simulink model "FLPD"  (R2024b)
settings: Solver=ode45  StartTime=0.0  StopTime=20  MinStep=0.00002  RelTol=1e-9
InitFcn:
  | addpath('./../Robot Description/Robot Data Package/meshes/visual/')
  | addpath('./../Dynamics and Kinematics/')
  | 
  | % Controller Design
  | Design;
values from neighbouring files (symbols this model uses):
  Kd = 100000    [Design.m]
  Kp = 100000    [Design.m]
  qInitDM = [zeros(14, 1)]    [Design.m]
settings Model: Creator=Banaan  LastModifiedBy=Banaan

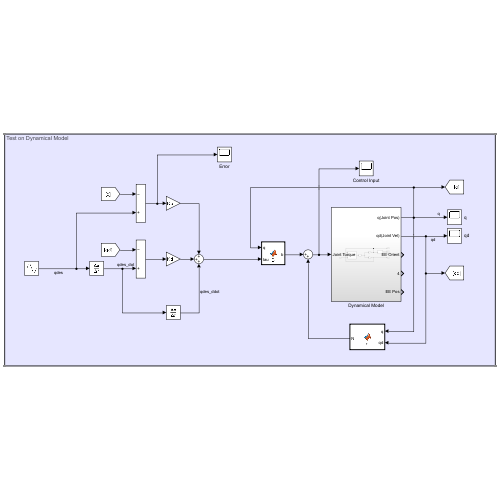
[thumbnail: Simulink's stored preview of the top-level diagram]
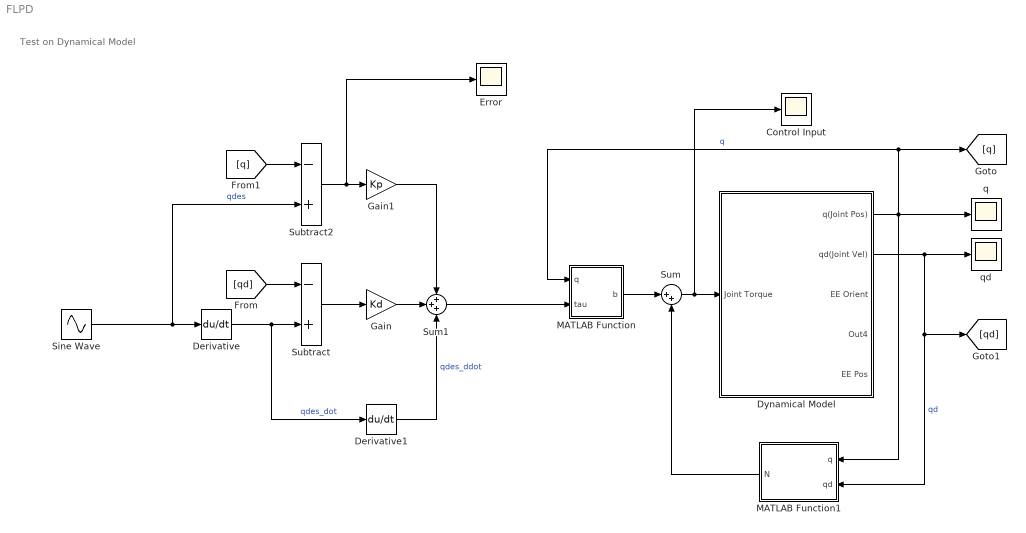
== system FLPD ==
  note: Test on Dynamical Model
  Control Input : Scope
  Derivative : Derivative
  Derivative1 : Derivative
  Dynamical Model : Subsystem
  Error : Scope
  Gain : Gain  Gain=Kd
  Gain1 : Gain  Gain=Kp
  MATLAB Function : MATLAB Function  TreatAsAtomicUnit=on
  MATLAB Function1 : MATLAB Function  TreatAsAtomicUnit=on
  Sine Wave : Sin  SampleTime=0
  Subtract : Sum  Inputs=-+
  Subtract2 : Sum  Inputs=-+
  Sum : Sum  Inputs=|++
  Sum1 : Sum  Inputs=+++
  q : Scope
  qd : Scope
  wires:
  Dynamical Model/1(q(Joint Pos)) -> [q], MATLAB Function/1(q), q/1, MATLAB Function1/1(q)  "q"
  Dynamical Model/2(qd(Joint Vel)) -> [qd], MATLAB Function1/2(qd), qd/1  "qd"
  Sum/1 -> Control Input/1, Dynamical Model/1(Joint Torque)
  MATLAB Function/1(b) -> Sum/1
  MATLAB Function1/1(N) -> Sum/2
  Sine Wave/1 -> Subtract2/2, Derivative/1  "qdes"
  Sum1/1 -> MATLAB Function/2(tau)
  Derivative/1 -> Derivative1/1, Subtract/2  "qdes_dot"
  [qd] -> Subtract/1
  [q] -> Subtract2/1
  Derivative1/1 -> Sum1/3  "qdes_ddot"
  Subtract/1 -> Gain/1
  Gain/1 -> Sum1/2
  Subtract2/1 -> Error/1, Gain1/1
  Gain1/1 -> Sum1/1

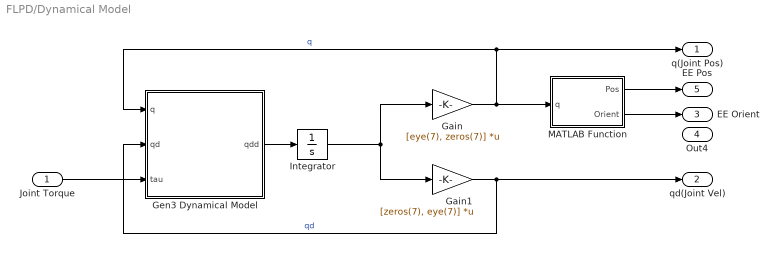
== system FLPD/Dynamical Model ==
  Joint Torque : Inport
  Gain : Gain  Gain=[eye(7), zeros(7)]  Multiplication=Matrix(K*u)
  Gain1 : Gain  Gain=[zeros(7), eye(7)]  Multiplication=Matrix(K*u)
  Gen3 Dynamical Model : MATLAB Function  TreatAsAtomicUnit=on
  Integrator : Integrator  InitialCondition=qInitDM
  MATLAB Function : MATLAB Function  TreatAsAtomicUnit=on
  q(Joint Pos) : Outport
  qd(Joint Vel) : Outport  Port=2
  EE Orient : Outport  Port=3
  Out4 : Outport  Port=4
  EE Pos : Outport  Port=5
  wires:
  Integrator/1 -> Gain/1, Gain1/1
  Gain/1 -> MATLAB Function/1(q), Gen3 Dynamical Model/1(q), q(Joint Pos)/1  "q"
  Gen3 Dynamical Model/1(qdd) -> Integrator/1
  Gain1/1 -> qd(Joint Vel)/1, Gen3 Dynamical Model/2(qd)  "qd"
  Joint Torque/1 -> Gen3 Dynamical Model/3(tau)
  MATLAB Function/1(Pos) -> EE Pos/1
  MATLAB Function/2(Orient) -> EE Orient/1

== matlab function FLPD/Dynamical Model/MATLAB Function ==
  data: q input; Pos output; Orient output
function [Pos, Orient] = FK(q) %#codegen
    coder.extrinsic('Gen3FK');

    tmp = zeros(6, 1);
    tmp = Gen3FK(q);

    Pos    = tmp(1:3, 1);
    Orient = tmp(4:6, 1);      % Order = [Yaw - Pitch - Roll]
end

== matlab function FLPD/MATLAB Function ==
  data: q input; b output; tau input
function b = B(q, tau) %#codegen
    coder.extrinsic('Gen3ODEFun_B');

    tmp = zeros(7, 7);
    tmp = Gen3ODEFun_B(q);

    b = zeros(7, 1);
    b = tmp * tau;
end

== matlab function FLPD/MATLAB Function1 ==
  data: q input; N output; qd input
function N = n(q, qd) %#codegen
    coder.extrinsic('Gen3ODEFun_C');
    coder.extrinsic('Gen3ODEFun_g');

    N = zeros(7, 1);
    C = zeros(7, 7);
    g = zeros(7, 1);
    
    C = Gen3ODEFun_C(q, qd);
    g = Gen3ODEFun_g(q);
    N = C * qd + g;
end

== matlab function FLPD/Dynamical Model/Gen3 Dynamical Model ==
  data: q input; qdd output; qd input; tau input
function qdd = fcn(q, qd, tau) %#codegen
    coder.extrinsic('Gen3ODEFun');

    qdd = zeros(14, 1);
    qdd = Gen3ODEFun(0, [q; qd], tau);
end
